simulink model "CompleteEngineModel_turbo"  (R2020a)
settings: Solver=ode23tb  StartTime=0  StopTime=600  MaxStep=0.4  RelTol=1e-6  AbsTol=1e-6  EnableMultiTasking=on
values from neighbouring files (symbols this model uses):
  A_eff_const = inv(A'*A)*A'*B    [Init_Project1.m]
  A_max_wg = 0.035^2/4*pi    (= 0.000962112750162)    [Init_Project1.m]    (also in Project2B.m = 0.000314159265359)
  AFs = EngineMap.airfuel.AFs    [Init_Project1.m]    (also in Project1b.m = 14)
  alpha_REF_manual = 0    [Init_Project1.m]    (also in Project2B.m)
  alphaEND = alphaINI    (= 0)    [Init_Project1.m]
  alphaINI = 0.0    (= 0)    [Init_Project1.m]
  alphaST = 30    [Init_Project1.m]
  Boost_control = 0    [Init_Project1.m]    (also in Project2B.m = 1)
  BSR_max = k(2)    [Project2A.m]
  C_d = x(3)    [Init_Project1.m]
  C_P0 = k(1)    [Project2A.m]
  C_P1 = k(2)    [Project2A.m]
  c_r1 = x(1)    [Init_Project1.m]
  c_r2 = x(2)    [Init_Project1.m]
  c_tc_fric = 1e-6    (= 1e-06)    [Init_Project1.m]    (also in Project2B.m)
  Cd_wg = 0.8    [Init_Project1.m]    (also in Project2B.m = 0.9)
  cp_air = gamma_air*cv_air    [Init_Project1.m]    (also in Project2A.m = 980)
  cp_exh = gamma_exh*cv_exh    [Init_Project1.m]    (also in Project2A.m = 1213.3)
  dP_thrREF = 10e3    (= 10000)    [Project2B.m]
  eta_c_max = k(1)    [Project2A.m]
  eta_t_max = k(1)    [Project2A.m]
  eta_vol_model = Intake_mainfold_const(1) + Intake_mainfold_const(2).*sqrt(p_im) + Intake_mainfold_const(3).*sqrt(N)    [Init_Project1.m]
  etaCmin = min(etaC/2)    [Project2A.m]
  etaTmin = min(turb.etaT)/2    [Project2A.m]
  Exhaust_flow_const = inv(A'*A)*A'*B    [Init_Project1.m]
  FMEP_const = inv(A'*A)*A'*B    [Init_Project1.m]
  Fuel_injection_const = inv(A'*A)*A'*B    [Init_Project1.m]
  gamma_air = EngineMap.airfuel.gamma_air    [Init_Project1.m]    (also in Project2A.m = 1.4)
  gamma_exh = EngineMap.airfuel.gamma_exh    [Init_Project1.m]    (also in Project2A.m = 1.3)
  Intake_mainfold_const = inv(A'*A)*A'*B    [Init_Project1.m]
  J_tc = 2.55e-5    (= 2.55e-05)    [Init_Project1.m]    (also in Project2B.m = 1e-05)
  k_0 = k(1)    [Project2A.m]
  k_1 = k(2)    [Project2A.m]
  KiDriver = 0.02    [Init_Project1.m]    (also in Project2B.m = 0.05)
  KpDriver = 0.04    [Init_Project1.m]    (also in Project2B.m = 0.8)
  KpThr = 1e-6    (= 1e-06)    [Init_Project1.m]    (also in Project2B.m)
  KpWg = 1e-6    (= 1e-06)    [Init_Project1.m]    (also in Project2B.m = 5e-06)
  m_dot_c_Corr_at = k(2)    [Project2A.m]
  m_dot_cCorr_max = k(2)    [Project2A.m]
  n_cyl = EngineMap.engine.n_cyl    [Init_Project1.m]    (also in Project2A.m)
  N_e_manual = 0    [Init_Project1.m]    (also in Project2B.m = 1)
  N_e_step = 1    [Init_Project1.m]    (also in Project2B.m)
  n_r = EngineMap.engine.n_r    [Init_Project1.m]    (also in Project2A.m; Project2B.m = 2)
  NEND = NINI    (= 2000)    [Init_Project1.m]    (also in Project2B.m = 2500)
  NeRampInit = 800    [Init_Project1.m]    (also in Project2B.m)
  NeSlope = 1    [Init_Project1.m]    (also in Project2B.m)
  NeST = 30    [Init_Project1.m]
  NINI = 2000    [Init_Project1.m]    (also in Project2B.m = 2500)
  p01 = comp.p01    [Project2A.m]
  p_amb = max(EngineMap.p_af)    [Init_Project1.m]
  pCref = comp.pCref    [Project2A.m]
  pedEND = 1.0    (= 1)    [Init_Project1.m]    (also in Project2B.m)
  pedINI = 0.2    [Init_Project1.m]    (also in Project2B.m = 0)
  pedPos_manual = 0    [Init_Project1.m]    (also in Project2B.m = 1)
  pedST = 30    [Init_Project1.m]    (also in Project2B.m)
  PiC_at = k(3)    [Project2A.m]
  Psi_max = k(1)    [Project2A.m]
  Q11 = k(4)    [Project2A.m]
  Q12 = k(5)    [Project2A.m]
  Q22 = k(6)    [Project2A.m]
  q_LHV = EngineMap.airfuel.q_LHV    [Init_Project1.m]
  R_air = EngineMap.airfuel.R_air    [Init_Project1.m]
  r_c = EngineMap.engine.r_c    [Init_Project1.m]    (also in Project1b.m = pCylHigh.r_c)
  R_exh = EngineMap.airfuel.R_exh    [Init_Project1.m]
  rComp = dComp/2    (= 0.028)    [Project2A.m]
  rho_air = p_amb/(R_air*T_amb)    [Init_Project1.m]
  rTurb = dTurb/2    (= 0.0261)    [Project2A.m]
  T01 = comp.T01    [Project2A.m]
  T_amb = mean(EngineMap.T_af)    [Init_Project1.m]
  T_bef_thr = EngineMap.T_bef_thr    [Init_Project1.m]
  T_es = EngineMap.T_es    [Init_Project1.m]
  T_ic = mean(T_bef_thr)    [Init_Project1.m]    (also in Project2B.m = T_im)
  T_im = EngineMap.T_im    [Init_Project1.m]    (also in Project1b.m = pCylHigh.T_im)
  tau_d = 0.069    [Init_Project1.m]
  tau_mix = 0.085    [Init_Project1.m]
  tau_th = 0.04    [Init_Project1.m]
  tau_wg = 0.1    [Init_Project1.m]    (also in Project2B.m)
  TCref = comp.TCref    [Project2A.m]
  Temp_const = inv(A'*A)*A'*B    [Init_Project1.m]
  TiThr = 0.1    [Init_Project1.m]    (also in Project2B.m = 0.4)
  TiWg = 4    [Init_Project1.m]    (also in Project2B.m = 7)
  V_D = EngineMap.engine.V_D    [Init_Project1.m]    (also in Project2B.m = n_cyl*V_d)
  V_d = 2*a*pi*B^2/4    [Init_Project1.m]    (also in Project2A.m; Project2B.m = B^2/4*pi*s)
  V_em = EngineMap.engine.V_em    [Init_Project1.m]
  V_es = EngineMap.engine.V_es    [Init_Project1.m]
  V_ic = 10e-3    (= 0.01)    [Init_Project1.m]    (also in Project2B.m)
  V_im = EngineMap.engine.V_im    [Init_Project1.m]
  VehicleArea = 2.0    (= 2)    [Init_Project1.m]
  VehicleMass = 1520    [Init_Project1.m]
  wg_REF_manual = 0    [Init_Project1.m]    (also in Project2B.m)
  wgEND = wgINI    (= 100)    [Init_Project1.m]
  wgINI = 100    [Init_Project1.m]
  wgST = 30    [Init_Project1.m]
  WheelRadius = 0.3    [Init_Project1.m]
undefined symbols (not defined in the file or in its folder): Newton, Raphson, TqEvsNe
libraries: simulink x2
(part 1 of 2)
settings Model: ExtModeTrigMode=oneshot  ExtModeArmWhenConnect=off  ExtModeAutoUpdateStatusClock=off  Creator=peran  LastModifiedBy=David Wiman
settings SolverCC: AutoScaleAbsTol=off
settings DataIOCC: SaveFormat=Array  SignalLoggingSaveFormat=ModelDataLogs  ReturnWorkspaceOutputs=off  SignalLoggingName=sigsOut
settings OptimizationCC: BlockReduction=off  BooleanDataType=off  ExpressionDepthLimit=2147483647  InitFltsAndDblsToZero=on  LifeSpan=inf
settings DebuggingCC: SaveWithParameterizedLinksMsg=none  UnderspecifiedInitializationDetection=Classic  MergeDetectMultiDrivingBlocksExec=none  SignalResolutionControl=TryResolveAllWithWarning  MultiTaskDSMMsg=warning  MultiTaskCondExecSysMsg=none  FcnCallInpInsideContextMsg=warning  StateNameClashWarn=warning  SFUnexpectedBacktrackingDiag=warning  SFNoUnconditionalDefaultTransitionDiag=warning  SFExecutionAtInitializationDiag=none  ArithmeticOperatorsInVariantConditions=warning
settings HardwareCC: ProdBitPerPointer=32  ProdBitPerSizeT=32  ProdBitPerPtrDiffT=32  ProdLargestAtomicFloat=None  ProdIntDivRoundTo=Undefined  ProdEndianess=Unspecified  ProdWordSize=32  ProdHWDeviceType=32-bit Generic  TargetUnknown=on
settings ModelReferenceCC: PropagateSignalLabelsOutOfModel=off
settings SFSimCC: SimUseLocalCustomCode=off  CustomCodeUndefinedFunction=UseInterfaceOnly
settings RTWCC: RTWUseLocalCustomCode=off
settings CodeAppCC: StateflowObjectComments=on
settings GRTTargetCC: TargetFcnLib=ansi_tfl_tmw.mat  TargetLangStandard=C89/C90 (ANSI)  ModelReferenceCompliant=off  CombineOutputUpdateFcns=off  MatFileLogging=off  GRTInterface=on
settings ConfigComp: CovMetricSettings=dw  CovHtmlReporting=on  CovSaveCumulativeToWorkspaceVar=on  CovSaveSingleToWorkspaceVar=on  CovExternalEMLEnable=off

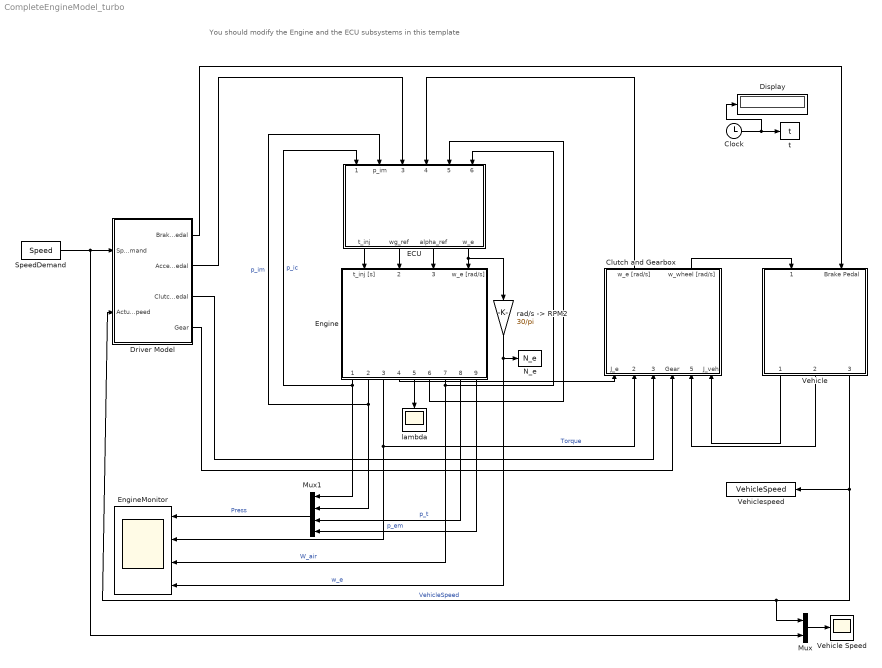
== system CompleteEngineModel_turbo ==
  note: You should modify the Engine and the ECU subsystems in this template
  Clock : Clock
  Clutch and Gearbox : Subsystem
  Display : Display
  Driver Model : Subsystem
  ECU : Subsystem
  Engine : Subsystem
  EngineMonitor : Scope  NumInputPorts=4
  Mux : Mux  Inputs=2
  Mux1 : Mux
  N_e : ToWorkspace  VariableName=N_e  SampleTime=-1
  SpeedDemand : FromWorkspace  VariableName=Speed  ZeroCross=off
  Vehicle : Subsystem
  Vehicle Speed : Scope
  Vehiclespeed : ToWorkspace  VariableName=VehicleSpeed  SampleTime=-1
  lambda : Scope
  "rad/s -> RPM2" : Gain  Gain=30/pi  SaturateOnIntegerOverflow=on  OutDataTypeStr=Inherit: Same as input  ParamDataTypeStr=Inherit: Same as input
  t : ToWorkspace  VariableName=t  SampleTime=-1
  wires:
  Vehicle/1(Vehicle Inertia [kgm^2]) -> Clutch and Gearbox/6(J_veh)
  Vehicle/2(Vehicle Torque [Nm]) -> Clutch and Gearbox/5(Tq_veh [Nm])
  Clutch and Gearbox/2(w_wheel [rad/s]) -> Vehicle/1(Wheel Speed [rad/s])
  Vehicle/3(Vehicle Speed[km/h]) -> Driver Model/2(Actual speed), Mux/1, Vehiclespeed/1  "VehicleSpeed"
  Driver Model/1(Brake Pedal) -> Vehicle/2(Brake Pedal)
  Driver Model/3(Clutch Pedal) -> Clutch and Gearbox/3(Clutch Pedal)
  Driver Model/2(Accelerator Pedal) -> ECU/3(ped_pos)
  Clutch and Gearbox/1(w_e [rad/s]) -> ECU/4(w_e [rad/s])
  SpeedDemand/1 -> Driver Model/1(Speed demand), Mux/2
  Driver Model/4(Gear) -> Clutch and Gearbox/4(Gear)
  Mux/1 -> Vehicle Speed/1
  Clock/1 -> t/1, Display/1
  Engine/7(m_dot_at [kg/s]) -> EngineMonitor/3, ECU/6(m_dot_air [kg/s])  "W_air"
  Engine/6(Lambda Disc) -> ECU/5(lambdaDisc)
  Engine/2(p_im [Pa]) -> Mux1/2, ECU/2(p_im)  "p_im"
  Engine/4(J_e [kgm^2]) -> Clutch and Gearbox/1(J_e)
  Engine/3(M_e [Nm]) -> EngineMonitor/2, Clutch and Gearbox/2(Tq_e [Nm])  "Torque"
  Engine/1(p_bef[Pa]) -> Mux1/1, ECU/1(p_ic [Pa])  "p_ic"
  Mux1/1 -> EngineMonitor/1  "Press"
  Engine/5(Lambda) -> lambda/1
  Engine/8(p_t [Pa]) -> Mux1/3  "p_t"
  Engine/9(p_em  [Pa]) -> Mux1/4  "p_em"
  ECU/4(w_e) -> "rad/s -> RPM2"/1, Engine/4(w_e [rad/s])
  "rad/s -> RPM2"/1 -> EngineMonitor/4, N_e/1  "w_e"
  ECU/2(wg_ref) -> Engine/2(wg_REF [0..1])
  ECU/3(alpha_ref) -> Engine/3(alpha_REF [0..1])
  ECU/1(t_inj) -> Engine/1(t_inj [s])

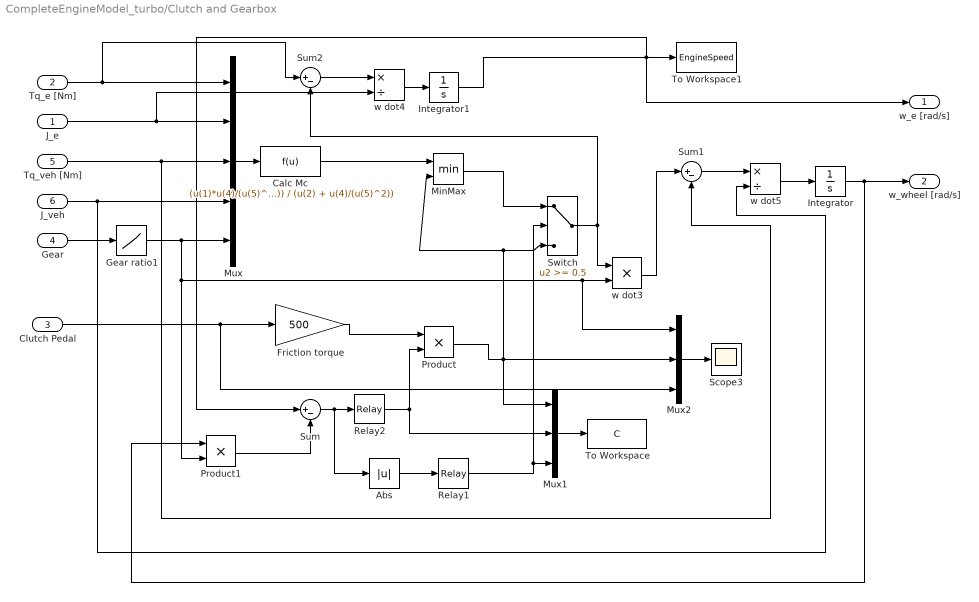
== system CompleteEngineModel_turbo/Clutch and Gearbox ==
  J_e : Inport
  Tq_e [Nm] : Inport  Port=2
  Clutch Pedal : Inport  Port=3
  Gear : Inport  Port=4
  Tq_veh [Nm] : Inport  Port=5
  J_veh : Inport  Port=6
  Abs : Abs  SaturateOnIntegerOverflow=on
  Calc Mc : Fcn  Expr=(u(1)*u(4)/(u(5)^2) + u(2)*u(3)/u(5)) / (u(2) + u(4)/(u(5)^2))
  Friction torque : Gain  Gain=500  SaturateOnIntegerOverflow=on  OutDataTypeStr=Inherit: Same as input  ParamDataTypeStr=Inherit: Same as input
  Gear ratio1 : Lookup  InputValues=[0:5]  Table=[30 16 7.5 4.5 3.2 2.5]  SaturateOnIntegerOverflow=on
  Integrator : Integrator
  Integrator1 : Integrator  InitialCondition=100  LimitOutput=on  LowerSaturationLimit=100
  MinMax : MinMax  Inputs=2  InputSameDT=on  SaturateOnIntegerOverflow=on
  Mux : Mux  Inputs=5
  Mux1 : Mux  Inputs=3
  Mux2 : Mux  Inputs=3
  Product : Product  InputSameDT=on  SaturateOnIntegerOverflow=on  OutDataTypeStr=Inherit: Same as first input
  Product1 : Product  InputSameDT=on  SaturateOnIntegerOverflow=on  OutDataTypeStr=Inherit: Same as first input
  Relay1 : Relay  OnSwitchValue=10  OffSwitchValue=1e-3  OnOutputValue=0  OffOutputValue=1
  Relay2 : Relay  OnSwitchValue=1e-1  OffSwitchValue=-1e-1  OffOutputValue=-1
  Scope3 : Scope
  Sum : Sum  Inputs=|+-  InputSameDT=on  SaturateOnIntegerOverflow=on  OutDataTypeStr=Inherit: Same as first input
  Sum1 : Sum  Inputs=|+-  InputSameDT=on  SaturateOnIntegerOverflow=on  OutDataTypeStr=Inherit: Same as first input
  Sum2 : Sum  Inputs=|+-  InputSameDT=on  SaturateOnIntegerOverflow=on  OutDataTypeStr=Inherit: Same as first input
  Switch : Switch  Threshold=0.5  SaturateOnIntegerOverflow=on  InputSameDT=on
  To Workspace : ToWorkspace  VariableName=C  SaveFormat=Structure With Time  SampleTime=-1
  To Workspace1 : ToWorkspace  VariableName=EngineSpeed  SaveFormat=Structure With Time  SampleTime=-1
  w dot3 : Product  Inputs=**  InputSameDT=on  SaturateOnIntegerOverflow=on  OutDataTypeStr=Inherit: Same as first input
  w dot4 : Product  Inputs=*/  InputSameDT=on  SaturateOnIntegerOverflow=on  OutDataTypeStr=Inherit: Same as first input
  w dot5 : Product  Inputs=*/  InputSameDT=on  SaturateOnIntegerOverflow=on  OutDataTypeStr=Inherit: Same as first input
  w_e [rad/s] : Outport
  w_wheel [rad/s] : Outport  Port=2
  wires:
  Switch/1 -> w dot3/1, Sum2/2
  Relay2/1 -> Mux1/2, Product/2
  Sum/1 -> Relay2/1, Abs/1
  Abs/1 -> Relay1/1
  MinMax/1 -> Switch/1
  Calc Mc/1 -> MinMax/1
  Mux/1 -> Calc Mc/1
  Mux2/1 -> Scope3/1
  Clutch Pedal/1 -> Friction torque/1, Mux2/3
  Tq_e [Nm]/1 -> Mux/1, Sum2/1
  J_e/1 -> Mux/2, w dot4/2
  Sum2/1 -> w dot4/1
  w dot4/1 -> Integrator1/1
  Integrator1/1 -> To Workspace1/1, w_e [rad/s]/1, Sum/1
  Relay1/1 -> Mux1/3, Switch/2
  Mux1/1 -> To Workspace/1
  Product1/1 -> Sum/2
  Product/1 -> MinMax/2, Switch/3, Mux2/2, Mux1/1
  Friction torque/1 -> Product/1
  Gear/1 -> Gear ratio1/1
  Gear ratio1/1 -> Product1/2, w dot3/2, Mux2/1, Mux/5
  w dot5/1 -> Integrator/1
  Sum1/1 -> w dot5/1
  Tq_veh [Nm]/1 -> Mux/3, Sum1/2
  J_veh/1 -> Mux/4, w dot5/2
  Integrator/1 -> w_wheel [rad/s]/1, Product1/1
  w dot3/1 -> Sum1/1

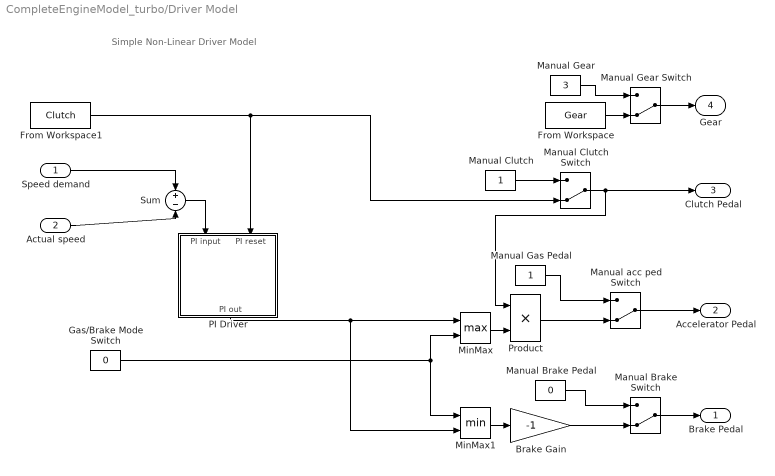
== system CompleteEngineModel_turbo/Driver Model ==
  note: Simple Non-Linear Driver Model
  Speed demand : Inport
  Actual speed : Inport  Port=2
  Brake Gain : Gain  Gain=-1  SaturateOnIntegerOverflow=on  OutDataTypeStr=Inherit: Same as input  ParamDataTypeStr=Inherit: Same as input
  From Workspace : FromWorkspace  VariableName=Gear  ZeroCross=off
  From Workspace1 : FromWorkspace  VariableName=Clutch  ZeroCross=off  OutputAfterFinalValue=Holding final value
  Gas/Brake Mode Switch : Constant  Value=0
  Manual Clutch : Constant
  Manual Gas Pedal : Constant
  Manual Gear : Constant  Value=3
  Manual Brake Pedal : Constant  Value=0
  Manual Brake Switch : ManualSwitch  CurrentSetting=0
  Manual Clutch Switch : ManualSwitch  CurrentSetting=0
  Manual Gear Switch : ManualSwitch  CurrentSetting=0
  Manual acc ped Switch : ManualSwitch  CurrentSetting=0
  MinMax : MinMax  Function=max  Inputs=2  InputSameDT=on  SaturateOnIntegerOverflow=on
  MinMax1 : MinMax  Inputs=2  InputSameDT=on  SaturateOnIntegerOverflow=on
  PI Driver : Subsystem
  Product : Product  InputSameDT=on  SaturateOnIntegerOverflow=on  OutDataTypeStr=Inherit: Same as first input
  Sum : Sum  Inputs=+-  InputSameDT=on  SaturateOnIntegerOverflow=on  OutDataTypeStr=Inherit: Same as first input
  Brake Pedal : Outport
  Accelerator Pedal : Outport  Port=2
  Clutch Pedal : Outport  Port=3
  Gear : Outport  Port=4
  wires:
  Product/1 -> Manual acc ped Switch/2
  MinMax/1 -> Product/2
  Manual acc ped Switch/1 -> Accelerator Pedal/1
  Manual Gas Pedal/1 -> Manual acc ped Switch/1
  Gas/Brake Mode Switch/1 -> MinMax1/1, MinMax/2
  MinMax1/1 -> Brake Gain/1
  PI Driver/1(PI out) -> MinMax1/2, MinMax/1
  From Workspace1/1 -> Manual Clutch Switch/2, PI Driver/2(PI reset)
  Manual Gear/1 -> Manual Gear Switch/1
  From Workspace/1 -> Manual Gear Switch/2
  Manual Gear Switch/1 -> Gear/1
  Manual Clutch/1 -> Manual Clutch Switch/1
  Brake Gain/1 -> Manual Brake Switch/2
  Manual Brake Pedal/1 -> Manual Brake Switch/1
  Manual Brake Switch/1 -> Brake Pedal/1
  Manual Clutch Switch/1 -> Clutch Pedal/1, Product/1
  Speed demand/1 -> Sum/1
  Sum/1 -> PI Driver/1(PI input)
  Actual speed/1 -> Sum/2

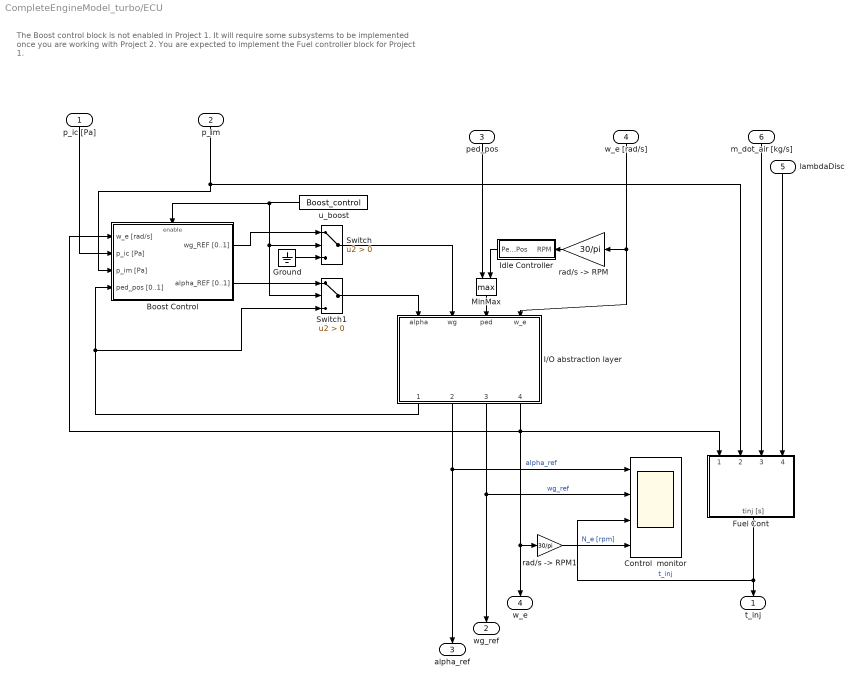
== system CompleteEngineModel_turbo/ECU ==
  note: The Boost control block is not enabled in Project 1. It will require some subsystems to be
      | implemented once you are working with Project 2.
      | You are expected to implement the Fuel controller block for Project 1.
  p_ic [Pa] : Inport
  p_im : Inport  Port=2
  ped_pos : Inport  Port=3
  w_e [rad/s] : Inport  Port=4
  lambdaDisc : Inport  Port=5
  m_dot_air [kg/s] : Inport  Port=6
  Boost Control : Subsystem
  Control  monitor : Scope  NumInputPorts=4
  Fuel Cont : Subsystem
  Ground : Ground
  I/O abstraction layer : Subsystem
  Idle Controller : Subsystem
  MinMax : MinMax  Function=max  Inputs=2  InputSameDT=on  SaturateOnIntegerOverflow=on
  Switch : Switch  Criteria=u2 > Threshold
  Switch1 : Switch  Criteria=u2 > Threshold
  "rad/s -> RPM" : Gain  Gain=30/pi  SaturateOnIntegerOverflow=on  OutDataTypeStr=Inherit: Same as input  ParamDataTypeStr=Inherit: Same as input
  "rad/s -> RPM1" : Gain  Gain=30/pi  SaturateOnIntegerOverflow=on  OutDataTypeStr=Inherit: Same as input  ParamDataTypeStr=Inherit: Same as input
  u_boost : Constant  Value=Boost_control
  t_inj : Outport
  wg_ref : Outport  Port=2
  alpha_ref : Outport  Port=3
  w_e : Outport  Port=4
  wires:
  Idle Controller/1(PedalPos) -> MinMax/2
  MinMax/1 -> I/O abstraction layer/3(ped)
  I/O abstraction layer/4(w_e [rad/s]) -> Boost Control/1("w_e [rad/s] "), Fuel Cont/1(w_e [rad/s]), w_e/1, "rad/s -> RPM1"/1
  w_e [rad/s]/1 -> I/O abstraction layer/4(w_e), "rad/s -> RPM"/1
  m_dot_air [kg/s]/1 -> Fuel Cont/3(m_dot_air [kg/s])
  p_ic [Pa]/1 -> Boost Control/2(p_ic [Pa])
  ped_pos/1 -> MinMax/1
  Fuel Cont/1(tinj [s]) -> Control  monitor/3, t_inj/1  "t_inj"
  I/O abstraction layer/2(alpha_REF [0..1]) -> Control  monitor/1, alpha_ref/1  "alpha_ref"
  I/O abstraction layer/3(wg_REF [0..100]) -> Control  monitor/2, wg_ref/1  "wg_ref"
  lambdaDisc/1 -> Fuel Cont/4(lambdaDisc)
  p_im/1 -> Boost Control/3(p_im [Pa]), Fuel Cont/2(p_im [Pa])
  "rad/s -> RPM"/1 -> Idle Controller/1(RPM)
  I/O abstraction layer/1(pedPos [0..1]) -> Boost Control/4(ped_pos [0..1]), Switch1/3
  u_boost/1 -> Boost Control/Enable, Switch1/2, Switch/2
  Boost Control/2(alpha_REF [0..1]) -> Switch1/1
  Switch1/1 -> I/O abstraction layer/1(alpha)
  Switch/1 -> I/O abstraction layer/2(wg)
  Boost Control/1(wg_REF [0..1]) -> Switch/1
  Ground/1 -> Switch/3
  "rad/s -> RPM1"/1 -> Control  monitor/4  "N_e [rpm]"

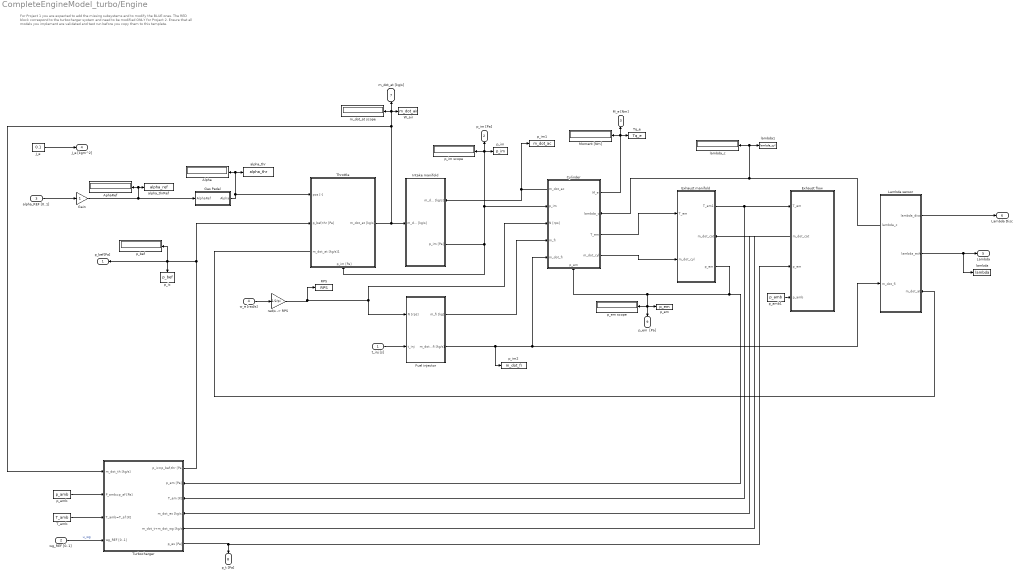
== system CompleteEngineModel_turbo/Engine ==
  note: For Project 1 you are expected to add the missing subsystems and to modify the BLUE ones.
      | The RED block correspond to the turbocharger system and need to be modified ONLY for Project 2.
      | Ensure that all models you implement are validated and test run before you copy them to this template.
  t_inj [s] : Inport
  wg_REF [0..1] : Inport  Port=2
  alpha_REF [0..1] : Inport  Port=3
  w_e [rad/s] : Inport  Port=4
  Alpha : Display
  AphaRef : Display
  Cylinder : Subsystem
      settings: PortSchema="{\"entries\":[{\"content\":{\"sides\":[{\"content\":{\"connectorIds\":[\"Out2\",\"Out3\",\"In1\",\"Out4\"]},\"type\":\"ConnectorPlacement.EquallySpacedRectSide\",\"uuid\":\"c6ff6295-f90b-4986-ac7a-70e0bce22d1f\"},{\"content\":{\"connectorIds\":[\"In3\",\"In4\",\"In5\",\"In6\",\"Out1\"],\"side\":\"RIGHT\"},\"type\":\"ConnectorPlacement.EquallySpacedRectSide\",\"uuid\":\"f8bbf01b-018f-4b58-b1b8-37d8ef2a501b\"},{\"content\":{\"connectorIds\":[\"In2\"],\"side\":\"TOP\"},\"type\":\"ConnectorPlacement.EquallySpacedRectSide\",\"uuid\":\"590f1776-0b6e-490b-9b82-c6a1f0298d63\"},{\"content\":{\"connectorIds\":[],\"side\":\"BOTTOM\"},\"type\":\"ConnectorPlacement.EquallySpacedRectSide\",\"uuid\":\"6fcd95e2-2788-44a0-9284-05f8c21997a1\"}]},\"type\":\"ConnectorPlacement.EquallySpacedConnector\",\"uuid\":\"69b978e9-63f0-4790-9255-9c73cc49e7a8\"}],\"packageUris\":[\"http://schema.mathworks.com/mf0/Connector/19700101\"],\"version\":\"1.0\"}"
  Exhaust flow : Subsystem
      settings: PortSchema="{\"entries\":[{\"content\":{\"sides\":[{\"content\":{\"connectorIds\":[\"In1\",\"Out1\",\"In2\",\"In3\"]},\"type\":\"ConnectorPlacement.EquallySpacedRectSide\",\"uuid\":\"f06335af-0d46-453e-89a7-85820e5b30b4\"},{\"content\":{\"connectorIds\":[],\"side\":\"RIGHT\"},\"type\":\"ConnectorPlacement.EquallySpacedRectSide\",\"uuid\":\"1980f551-ae72-440d-afc1-b2b6b725f391\"},{\"content\":{\"connectorIds\":[],\"side\":\"TOP\"},\"type\":\"ConnectorPlacement.EquallySpacedRectSide\",\"uuid\":\"7f9d811b-4ba7-47b4-9941-e90fdf29edc9\"}]},\"type\":\"ConnectorPlacement.EquallySpacedConnector\",\"uuid\":\"d9ed9e77-87d7-4fb4-9a8b-d019adccfd00\"}],\"packageUris\":[\"http://schema.mathworks.com/mf0/Connector/19700101\"],\"version\":\"1.0\"}"
  Exhaust manifold : Subsystem
      settings: PortSchema="{\"entries\":[{\"content\":{\"sides\":[{\"content\":{\"connectorIds\":[\"In1\",\"In2\"]},\"type\":\"ConnectorPlacement.EquallySpacedRectSide\",\"uuid\":\"ecdbb782-eef7-477e-bb82-5ebf032163a3\"},{\"content\":{\"connectorIds\":[\"Out1\",\"In3\",\"Out2\"],\"side\":\"RIGHT\"},\"type\":\"ConnectorPlacement.EquallySpacedRectSide\",\"uuid\":\"4b5fba5e-4300-4916-aa15-d3f6c61d9689\"},{\"content\":{\"connectorIds\":[],\"side\":\"TOP\"},\"type\":\"ConnectorPlacement.EquallySpacedRectSide\",\"uuid\":\"210fa4c6-63e4-484e-b7fb-4f2899d71e64\"}]},\"type\":\"ConnectorPlacement.EquallySpacedConnector\",\"uuid\":\"ab4f6bcc-96c1-47e6-9038-ce7b6e5d4830\"}],\"packageUris\":[\"http://schema.mathworks.com/mf0/Connector/19700101\"],\"version\":\"1.0\"}"
  Fuel injector : Subsystem
      settings: PortSchema="{\"entries\":[{\"content\":{\"sides\":[{\"content\":{\"connectorIds\":[]},\"type\":\"ConnectorPlacement.EquallySpacedRectSide\",\"uuid\":\"c6ff6295-f90b-4986-ac7a-70e0bce22d1f\"},{\"content\":{\"connectorIds\":[],\"side\":\"RIGHT\"},\"type\":\"ConnectorPlacement.EquallySpacedRectSide\",\"uuid\":\"f8bbf01b-018f-4b58-b1b8-37d8ef2a501b\"},{\"content\":{\"connectorIds\":[\"In1\",\"In2\"],\"side\":\"TOP\"},\"type\":\"ConnectorPlacement.EquallySpacedRectSide\",\"uuid\":\"590f1776-0b6e-490b-9b82-c6a1f0298d63\"},{\"content\":{\"connectorIds\":[\"Out1\",\"Out2\"],\"side\":\"BOTTOM\"},\"type\":\"ConnectorPlacement.EquallySpacedRectSide\",\"uuid\":\"6fcd95e2-2788-44a0-9284-05f8c21997a1\"}]},\"type\":\"ConnectorPlacement.EquallySpacedConnector\",\"uuid\":\"69b978e9-63f0-4790-9255-9c73cc49e7a8\"}],\"packageUris\":[\"http://schema.mathworks.com/mf0/Connector/19700101\"],\"version\":\"1.0\"}"
  Gain : Gain
  Gas Pedal : Subsystem
  Intake manifold : Subsystem
      settings: PortSchema="{\"entries\":[{\"content\":{\"sides\":[{\"content\":{\"connectorIds\":[\"In1\"]},\"type\":\"ConnectorPlacement.EquallySpacedRectSide\",\"uuid\":\"c4e4d620-2bcc-4db0-9055-5904ec1a58a9\"},{\"content\":{\"connectorIds\":[\"In2\",\"Out1\"],\"side\":\"RIGHT\"},\"type\":\"ConnectorPlacement.EquallySpacedRectSide\",\"uuid\":\"7abafa54-675f-4448-8d24-7b3f9f41fe2d\"},{\"content\":{\"connectorIds\":[],\"side\":\"TOP\"},\"type\":\"ConnectorPlacement.EquallySpacedRectSide\",\"uuid\":\"2b3cebc2-f79e-4be9-b6ba-c95bab7e4fe0\"}]},\"type\":\"ConnectorPlacement.EquallySpacedConnector\",\"uuid\":\"07f49e90-8b24-4894-a061-cd1894b00575\"}],\"packageUris\":[\"http://schema.mathworks.com/mf0/Connector/19700101\"],\"version\":\"1.0\"}"
  J_e : Constant  Value=0.1
  Lambda sensor : Subsystem
      settings: PortSchema="{\"entries\":[{\"content\":{\"sides\":[{\"content\":{\"connectorIds\":[\"Out3\",\"In1\"]},\"type\":\"ConnectorPlacement.EquallySpacedRectSide\",\"uuid\":\"d39da2a0-5083-429f-b2a5-f3c55751e588\"},{\"content\":{\"connectorIds\":[\"Out1\",\"Out2\",\"In2\"],\"side\":\"RIGHT\"},\"type\":\"ConnectorPlacement.EquallySpacedRectSide\",\"uuid\":\"7673ed93-c321-42ef-ae67-bddda5587c96\"},{\"content\":{\"connectorIds\":[],\"side\":\"TOP\"},\"type\":\"ConnectorPlacement.EquallySpacedRectSide\",\"uuid\":\"0618fb4e-cce3-4388-971c-f8e6f06df9e4\"}]},\"type\":\"ConnectorPlacement.EquallySpacedConnector\",\"uuid\":\"03a84aa5-1ec4-4792-999b-2db4677b5033\"}],\"packageUris\":[\"http://schema.mathworks.com/mf0/Connector/19700101\"],\"version\":\"1.0\"}"
  Moment [Nm] : Display
  RPS : ToWorkspace  VariableName=RPS  SampleTime=-1
  T_amb : Constant  Value=T_amb
  "Throttle " : Subsystem
      settings: PortSchema="{\"entries\":[{\"content\":{\"sides\":[{\"content\":{\"connectorIds\":[\"Out2\"]},\"type\":\"ConnectorPlacement.EquallySpacedRectSide\",\"uuid\":\"c928f7f6-9f01-47f3-9bc0-46ff39781eb1\"},{\"content\":{\"connectorIds\":[\"In2\",\"In3\",\"Out1\"],\"side\":\"RIGHT\"},\"type\":\"ConnectorPlacement.EquallySpacedRectSide\",\"uuid\":\"8dd06eba-1f93-4a48-ba14-c22296a753f6\"},{\"content\":{\"connectorIds\":[],\"side\":\"TOP\"},\"type\":\"ConnectorPlacement.EquallySpacedRectSide\",\"uuid\":\"bb338683-60ae-4c40-9ad3-c06e2955afea\"},{\"content\":{\"connectorIds\":[\"In1\"],\"side\":\"BOTTOM\"},\"type\":\"ConnectorPlacement.EquallySpacedRectSide\",\"uuid\":\"0777e4e3-014c-463e-89e2-078be8dd0ff9\"}]},\"type\":\"ConnectorPlacement.EquallySpacedConnector\",\"uuid\":\"cbd452b7-e40d-41fa-8c5f-0189a331593c\"}],\"packageUris\":[\"http://schema.mathworks.com/mf0/Connector/19700101\"],\"version\":\"1.0\"}"
  Tq_e : ToWorkspace  VariableName=Tq_e  SampleTime=-1
  Turbocharger : Subsystem
      settings: PortSchema="{\"entries\":[{\"content\":{\"sides\":[{\"content\":{\"connectorIds\":[\"In1\",\"In2\",\"In3\",\"In4\"]},\"type\":\"ConnectorPlacement.EquallySpacedRectSide\",\"uuid\":\"86731332-f34d-46da-85bd-bb4bed14e334\"},{\"content\":{\"connectorIds\":[\"Out1\",\"In5\",\"In6\",\"In7\",\"Out2\",\"Out3\"],\"side\":\"RIGHT\"},\"type\":\"ConnectorPlacement.EquallySpacedRectSide\",\"uuid\":\"d31b5450-3593-487b-907f-2875749d4d92\"},{\"content\":{\"connectorIds\":[],\"side\":\"TOP\"},\"type\":\"ConnectorPlacement.EquallySpacedRectSide\",\"uuid\":\"0bb27454-71b6-4622-a06e-14bed29e19cf\"}]},\"type\":\"ConnectorPlacement.EquallySpacedConnector\",\"uuid\":\"668c2a51-25ad-4723-a90c-4999ba09b381\"}],\"packageUris\":[\"http://schema.mathworks.com/mf0/Connector/19700101\"],\"version\":\"1.0\"}"
  W_air : ToWorkspace  VariableName=m_dot_air  SampleTime=-1
  alpha_thr : ToWorkspace  VariableName=alpha_thr  SampleTime=-1
  alpha_thrRef : ToWorkspace  VariableName=alpha_ref  SampleTime=-1
  lambda : ToWorkspace  VariableName=lambda  SampleTime=-1
  lambda1 : ToWorkspace  VariableName=lambda_cyl  SampleTime=-1
  lambda_c : Display
  m_dot_at scope : Display
  p_amb : Constant  Value=p_amb
  p_amb1 : Constant  Value=p_amb
  p_bef : Display
  p_em : ToWorkspace  VariableName=p_em  SampleTime=-1
  p_em scope : Display
  p_ic : ToWorkspace  VariableName=p_bef  SampleTime=-1
  p_im : ToWorkspace  VariableName=p_im  SampleTime=-1
  p_im scope : Display
  p_im1 : ToWorkspace  VariableName=m_dot_ac  SampleTime=-1
  p_im2 : ToWorkspace  VariableName=m_dot_fi  SampleTime=-1
  "rad/s -> RPS" : Gain  Gain=1/2/pi  SaturateOnIntegerOverflow=on  OutDataTypeStr=Inherit: Same as input  ParamDataTypeStr=Inherit: Same as input
  p_bef[Pa] : Outport
  p_im [Pa] : Outport  Port=2
  M_e [Nm] : Outport  Port=3
  J_e [kgm^2] : Outport  Port=4
  Lambda : Outport  Port=5
  Lambda Disc : Outport  Port=6
  m_dot_at [kg/s] : Outport  Port=7
  p_t [Pa] : Outport  Port=8
  p_em  [Pa] : Outport  Port=9
  wires:
  J_e/1 -> J_e [kgm^2]/1
  Gas Pedal/1(Alpha) -> Alpha/1, alpha_thr/1, "Throttle "/2(pos [-])
  Lambda sensor/2(lambda_exh) -> Lambda/1, lambda/1
  Lambda sensor/1(lambda_disc) -> Lambda Disc/1
  wg_REF [0..1]/1 -> Turbocharger/4(wg_REF [0..1])  "u_wg"
  Turbocharger/3(p_es [Pa]) -> Exhaust flow/2(p_em), p_t [Pa]/1
  Turbocharger/1(p_ic=p_bef,thr [Pa]) -> "Throttle "/3(p_bef,thr [Pa]), p_bef/1, p_ic/1, p_bef[Pa]/1
  Fuel injector/2(m_fi [kg]) -> Cylinder/4(m_fi)
  Fuel injector/1(m_dot_fi [kg/s]) -> p_im2/1, Lambda sensor/1(m_dot_fi), Cylinder/3(m_dot_fi)
  Exhaust flow/1(m_dot_cat) -> Turbocharger/7(m_dot_es [kg/s])
  p_amb1/1 -> Exhaust flow/3(p_amb)
  Cylinder/1(m_dot_ac) -> p_im1/1, Intake manifold/2(m_dot_ac [kg/s])
  Gain/1 -> AphaRef/1, alpha_thrRef/1, Gas Pedal/1(AlphaRef)
  "rad/s -> RPS"/1 -> RPS/1, Fuel injector/2(N [rps]), Cylinder/5(N [rps])
  t_inj [s]/1 -> Fuel injector/1(t_inj)
  Intake manifold/1(p_im [Pa]) -> p_im/1, p_im scope/1, p_im [Pa]/1, Cylinder/6(p_im), "Throttle "/1(p_im [Pa])
  "Throttle "/2(m_dot_at [kg/s]) -> W_air/1, m_dot_at scope/1, m_dot_at [kg/s]/1, Turbocharger/1(m_dot_th [kg/s]), Intake manifold/1(m_dot_at [kg/s])
  Cylinder/4(M_e) -> Moment [Nm]/1, M_e [Nm]/1, Tq_e/1
  Cylinder/2(m_dot_cyl) -> Exhaust manifold/2(m_dot_cyl)
  Cylinder/3(T_em) -> Exhaust manifold/1(T_em)
  Exhaust manifold/1(T_em1) -> Turbocharger/6(T_em [K]), Exhaust flow/1(T_em)
  Exhaust manifold/2(p_em) -> Turbocharger/5(p_em [Pa]), p_em/1, p_em scope/1, p_em  [Pa]/1, Cylinder/2(p_em)
  Lambda sensor/3(lambda_c) -> lambda1/1, lambda_c/1, Cylinder/1(lambda_c)
  "Throttle "/1(m_dot_at [kg/s]1) -> Lambda sensor/2(m_dot_at)
  alpha_REF [0..1]/1 -> Gain/1
  w_e [rad/s]/1 -> "rad/s -> RPS"/1
  T_amb/1 -> Turbocharger/3(T_amb=T_af [K])
  p_amb/1 -> Turbocharger/2("P_amb=p_af [Pa] ")
  Turbocharger/2(m_dot_t+m_dot_wg [kg/s]) -> Exhaust manifold/3(m_dot_cat)

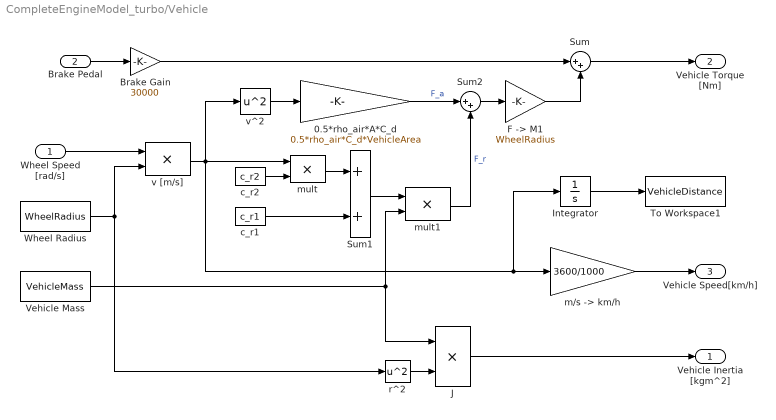
== system CompleteEngineModel_turbo/Vehicle ==
  Wheel Speed [rad/s] : Inport
  Brake Pedal : Inport  Port=2
  0.5*rho_air*A*C_d : Gain  Gain=0.5*rho_air*C_d*VehicleArea  SaturateOnIntegerOverflow=on  OutDataTypeStr=Inherit: Same as input  ParamDataTypeStr=Inherit: Same as input
  Brake Gain : Gain  Gain=30000  SaturateOnIntegerOverflow=on  OutDataTypeStr=Inherit: Same as input  ParamDataTypeStr=Inherit: Same as input
  "F -> M1" : Gain  Gain=WheelRadius  SaturateOnIntegerOverflow=on  OutDataTypeStr=Inherit: Same as input  ParamDataTypeStr=Inherit: Same as input
  Integrator : Integrator
  J : Product  SaturateOnIntegerOverflow=on  OutDataTypeStr=Inherit: Same as first input
  Sum : Sum  Inputs=|++  SaturateOnIntegerOverflow=on
  Sum1 : Sum  SaturateOnIntegerOverflow=on
  Sum2 : Sum  Inputs=|++  SaturateOnIntegerOverflow=on
  To Workspace1 : ToWorkspace  VariableName=VehicleDistance  SampleTime=-1
  Vehicle Mass : Constant  Value=VehicleMass
  Wheel Radius : Constant  Value=WheelRadius
  c_r1 : Constant  Value=c_r1
  c_r2 : Constant  Value=c_r2
  "m/s -> km/h" : Gain  Gain=3600/1000  SaturateOnIntegerOverflow=on  OutDataTypeStr=Inherit: Same as input  ParamDataTypeStr=Inherit: Same as input
  mult : Product  SaturateOnIntegerOverflow=on  OutDataTypeStr=Inherit: Same as first input
  mult1 : Product  SaturateOnIntegerOverflow=on  OutDataTypeStr=Inherit: Same as first input
  r^2 : Math  Operator=square  SignedPower=on  SaturateOnIntegerOverflow=on
  v [m/s] : Product  SaturateOnIntegerOverflow=on  OutDataTypeStr=Inherit: Same as first input
  v^2 : Math  Operator=square  SignedPower=on  SaturateOnIntegerOverflow=on
  Vehicle Inertia [kgm^2] : Outport
  Vehicle Torque [Nm] : Outport  Port=2
  Vehicle Speed[km/h] : Outport  Port=3
  wires:
  Brake Pedal/1 -> Brake Gain/1
  Wheel Radius/1 -> v [m/s]/2, r^2/1
  v [m/s]/1 -> Integrator/1, "m/s -> km/h"/1, mult/1, v^2/1
  "m/s -> km/h"/1 -> Vehicle Speed[km/h]/1
  Brake Gain/1 -> Sum/1
  Sum/1 -> Vehicle Torque [Nm]/1
  r^2/1 -> J/2
  Vehicle Mass/1 -> mult1/2, J/1
  J/1 -> Vehicle Inertia [kgm^2]/1
  Integrator/1 -> To Workspace1/1
  Wheel Speed [rad/s]/1 -> v [m/s]/1
  c_r2/1 -> mult/2
  mult/1 -> Sum1/1
  c_r1/1 -> Sum1/2
  Sum1/1 -> mult1/1
  mult1/1 -> Sum2/2  "F_r"
  v^2/1 -> 0.5*rho_air*A*C_d/1
  0.5*rho_air*A*C_d/1 -> Sum2/1  "F_a"
  Sum2/1 -> "F -> M1"/1
  "F -> M1"/1 -> Sum/2

== system CompleteEngineModel_turbo/Driver Model/PI Driver ==
  PI input : Inport
  PI reset : Inport  Port=2
  Integrator : Integrator  ExternalReset=either  LimitOutput=on  UpperSaturationLimit=30  LowerSaturationLimit=0
  Ki : Gain  Gain=KiDriver  SaturateOnIntegerOverflow=on  OutDataTypeStr=Inherit: Same as input  ParamDataTypeStr=Inherit: Same as input
  Kp : Gain  Gain=KpDriver  SaturateOnIntegerOverflow=on  OutDataTypeStr=Inherit: Same as input  ParamDataTypeStr=Inherit: Same as input
  Saturation : Saturate  UpperLimit=1  LowerLimit=-1
  Sum : Sum  Inputs=|++  InputSameDT=on  SaturateOnIntegerOverflow=on  OutDataTypeStr=Inherit: Same as first input
  PI out : Outport
  wires:
  PI input/1 -> Kp/1, Integrator/1
  Integrator/1 -> Ki/1
  Ki/1 -> Sum/2
  Sum/1 -> Saturation/1
  Saturation/1 -> PI out/1
  PI reset/1 -> Integrator/2
  Kp/1 -> Sum/1

== system CompleteEngineModel_turbo/ECU/Boost Control ==
  note: For Project 2 , the diver gas pedal interpretation and the throttle feed forward blocks need to be implemented.
  "w_e [rad/s] " : Inport
  p_ic [Pa] : Inport  Port=2
  p_im [Pa] : Inport  Port=3
  ped_pos [0..1] : Inport  Port=4
  Enable : EnablePort
  Constant : Constant  Value=0
  Constant1 : Constant
  Driver gas pedal interpretation : Subsystem
  Subtract1 : Sum
  Throttle saturation [0..1] : Saturate  UpperLimit=1  LowerLimit=0
  "Throttle Feed Forward " : Subsystem
  Throttle Feedback including anti-windup : Subsystem
  Waste-gate saturation [0..1] : Saturate  UpperLimit=1  LowerLimit=0
  Waste-gate Feedback including anti-windup1 : Subsystem
  "rad/s -> rpm" : Gain  Gain=30/pi  SaturateOnIntegerOverflow=on  OutDataTypeStr=Inherit: Same as input  ParamDataTypeStr=Inherit: Same as input
  thr_feedback_switch : ManualSwitch
  wg_feedback_switch : ManualSwitch
  wg_REF [0..1] : Outport
  alpha_REF [0..1] : Outport  Port=2
  wires:
  "Throttle Feed Forward "/1(alpha_thrFF [0..1]) -> Subtract1/1
  Throttle Feedback including anti-windup/1(alpha_thrFB [0..1]) -> thr_feedback_switch/1
  Subtract1/1 -> Throttle saturation [0..1]/1, Throttle Feedback including anti-windup/4(alpha_thrREF [0..1])
  "rad/s -> rpm"/1 -> "Throttle Feed Forward "/2(N_e [rpm]), Driver gas pedal interpretation/2(N_e [rpm])
  Throttle saturation [0..1]/1 -> alpha_REF [0..1]/1, Throttle Feedback including anti-windup/3(alpha_thrREFsat [0..1])
  Waste-gate saturation [0..1]/1 -> wg_REF [0..1]/1, Waste-gate Feedback including anti-windup1/3(wgREFsat [0..1])
  "w_e [rad/s] "/1 -> "rad/s -> rpm"/1
  p_ic [Pa]/1 -> Waste-gate Feedback including anti-windup1/2(p_icACT [Pa]), "Throttle Feed Forward "/3(p_icACT [Pa])
  p_im [Pa]/1 -> Throttle Feedback including anti-windup/2(p_imACT [Pa])
  Driver gas pedal interpretation/1(p_im_ref) -> "Throttle Feed Forward "/1(p_imREF [Pa]), Throttle Feedback including anti-windup/1(p_imREF [Pa])
  Driver gas pedal interpretation/2(p_ic_ref) -> Waste-gate Feedback including anti-windup1/1(p_icREF [Pa])
  Constant/1 -> thr_feedback_switch/2
  thr_feedback_switch/1 -> Subtract1/2
  ped_pos [0..1]/1 -> Driver gas pedal interpretation/1(ped_pos [0..1])
  Waste-gate Feedback including anti-windup1/1(wgFB [0..1]) -> wg_feedback_switch/1, Waste-gate Feedback including anti-windup1/4(wgREF [0..1])
  Constant1/1 -> wg_feedback_switch/2
  wg_feedback_switch/1 -> Waste-gate saturation [0..1]/1

== system CompleteEngineModel_turbo/ECU/Fuel Cont ==
  note: You have to implement here your fuel controller
  w_e [rad/s] : Inport
  p_im [Pa] : Inport  Port=2
  m_dot_air [kg/s] : Inport  Port=3
  lambdaDisc : Inport  Port=4
  Constant1 : Constant
  Divide1 : Product  Inputs=*/
  Gain : Gain  Gain=1/AFs
  Gain2 : Gain  Gain=n_r/(n_cyl*Fuel_injection_const(1))
  PID Controller : simulink/Continuous/PID Controller  Controller=PI  Form=Parallel  TimeDomain=Continuous-time  UseExternalTs=off  SampleTime=-1  IntegratorMethod=Forward Euler  FilterMethod=Forward Euler  ControllerParametersSource=internal  P=0.069*0.1/2  I=0.1  D=0.1  UseFilter=on  N=100  TunerSelectOption=Transfer Function Based (PID Tuner App)  InitialConditionSource=internal  InitialConditionForIntegrator=0  InitialConditionForFilter=0  DifferentiatorICPrevScaledInput=0  ExternalReset=none  TrackingMode=off  Kt=1  LimitOutput=off  UpperSaturationLimit=0.5  LowerSaturationLimit=-0.5  LinearizeAsGain=on  AntiWindupMode=none  Kb=1  POutMin=[]  POutMax=[]  IOutMin=[]  IOutMax=[]  DOutMin=[]  DOutMax=[]  NOutMin=[]  NOutMax=[]  SumOutMin=[]  SumOutMax=[]  SaturationOutMin=[]  SaturationOutMax=[]  PParamMin=[]  PParamMax=[]  IParamMin=[]  IParamMax=[]  DParamMin=[]  DParamMax=[]  NParamMin=[]  NParamMax=[]  KbParamMin=[]  KbParamMax=[]  KtParamMin=[]  KtParamMax=[]  KbOutMin=[]  KbOutMax=[]  KtOutMin=[]  KtOutMax=[]  IntegratorOutMin=[]  IntegratorOutMax=[]  FilterOutMin=[]  FilterOutMax=[]  SumI1OutMin=[]  SumI1OutMax=[]  SumI2OutMin=[]  SumI2OutMax=[]  SumI3OutMin=[]  SumI3OutMax=[]  SumI4OutMin=[]  SumI4OutMax=[]  SumDOutMin=[]  SumDOutMax=[]  DifferentiatorOutMin=[]  DifferentiatorOutMax=[]  FilterDiffOutCoefMin=[]  FilterDiffOutCoefMax=[]  ReciprocalOutMin=[]  ReciprocalOutMax=[]  SumDenOutMin=[]  SumDenOutMax=[]  SumNumOutMin=[]  SumNumOutMax=[]  DivideOutMin=[]  DivideOutMax=[]  UdiffTsProdOutMin=[]  UdiffTsProdOutMax=[]  NTsProdOutMin=[]  NTsProdOutMax=[]  UintegralTsProdOutMin=[]  UintegralTsProdOutMax=[]  UngainTsProdOutMin=[]  UngainTsProdOutMax=[]  IntegratorContinuousStateAttributes=''  IntegratorStateMustResolveToSignalObject=off  IntegratorRTWStateStorageClass=Auto  FilterContinuousStateAttributes=''  FilterStateMustResolveToSignalObject=off  FilterRTWStateStorageClass=Auto  ParallelPVariant=InternalParameters  IdealPVariant=Disabled  IVariant=InternalParameters  DVariant=Disabled  IntegratorVariant=Continuous  SatVariant=Disabled  AWVariant=Passthrough  PCopyVariant=Disabled  TRVariant=Disabled  FdbkBlocksVariant=Forward  IdealPFdbkVariant=Disabled  SatFdbkVariant=Disabled  DerivativeFilterVariant=Disabled  NVariant=Disabled  NCopyVariant=Disabled_SignalSpec  FilterICVariant=Disabled  IntegratorICVariant=InternalICs  ExternalResetVariant=Disabled  TRSumVariant=Passthrough  SumFdbkVariant=Disabled  SumVariant=Sum_PI  TsampFilterVariant=InternalTs  TsampNgainVariant=Passthrough  TsampIntegralVariant=Passthrough
  Product : Product
  Sum : Sum  Inputs=|++
  Sum1 : Sum  Inputs=|++
  Terminator1 : Terminator
  m_dot_ac_system : Subsystem
  "rad/s -> RPS" : Gain  Gain=1/2/pi  SaturateOnIntegerOverflow=on  OutDataTypeStr=Inherit: Same as input  ParamDataTypeStr=Inherit: Same as input
  t_0 : Constant  Value=Fuel_injection_const(2)
  tinj [s] : Outport
  wires:
  p_im [Pa]/1 -> m_dot_ac_system/1(p_im)
  lambdaDisc/1 -> PID Controller/1
  m_dot_ac_system/1(m_dot_ac) -> Gain/1
  Gain/1 -> Product/1
  m_dot_air [kg/s]/1 -> Terminator1/1
  Gain2/1 -> Divide1/1
  Divide1/1 -> Sum1/1
  t_0/1 -> Sum1/2
  Sum1/1 -> tinj [s]/1
  "rad/s -> RPS"/1 -> Divide1/2, m_dot_ac_system/2(N)
  PID Controller/1 -> Sum/1
  Constant1/1 -> Sum/2
  Product/1 -> Gain2/1
  w_e [rad/s]/1 -> "rad/s -> RPS"/1
  Sum/1 -> Product/2  "F_fc"

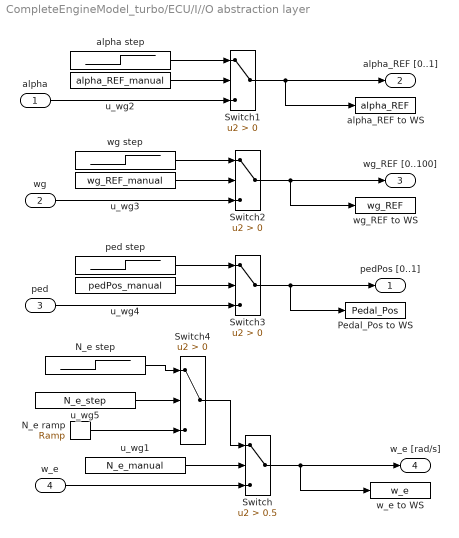
== system CompleteEngineModel_turbo/ECU/I//O abstraction layer ==
  alpha : Inport
  wg : Inport  Port=2
  ped : Inport  Port=3
  w_e : Inport  Port=4
  N_e ramp : simulink/Sources/Ramp  slope=NeSlope*pi/30  start=NeStartTime  InitialOutput=NeRampInit*pi/30
  N_e step : Step  Time=NeST  Before=NINI*pi/30  After=NEND*pi/30  SampleTime=0
  Pedal_Pos to WS : ToWorkspace  VariableName=Pedal_Pos  SampleTime=-1
  Switch : Switch  Criteria=u2 > Threshold  Threshold=0.5
  Switch{1..4} (4 alike) : Switch  Criteria=u2 > Threshold
  alpha step : Step  Time=alphaST  Before=alphaINI  After=alphaEND  SampleTime=0
  alpha_REF to WS : ToWorkspace  VariableName=alpha_REF  SampleTime=-1
  ped step : Step  Time=pedST  Before=pedINI  After=pedEND  SampleTime=0
  u_wg1 : Constant  Value=N_e_manual
  u_wg2 : Constant  Value=alpha_REF_manual
  u_wg3 : Constant  Value=wg_REF_manual
  u_wg4 : Constant  Value=pedPos_manual
  u_wg5 : Constant  Value=N_e_step
  w_e to WS : ToWorkspace  VariableName=w_e  SampleTime=-1
  wg step : Step  Time=wgST  Before=wgINI  After=wgEND  SampleTime=0
  wg_REF to WS : ToWorkspace  VariableName=wg_REF  SampleTime=-1
  pedPos [0..1] : Outport
  alpha_REF [0..1] : Outport  Port=2
  wg_REF [0..100] : Outport  Port=3
  w_e [rad/s] : Outport  Port=4
  wires:
  Switch/1 -> w_e [rad/s]/1, w_e to WS/1
  u_wg1/1 -> Switch/2
  w_e/1 -> Switch/3
  Switch1/1 -> alpha_REF [0..1]/1, alpha_REF to WS/1
  alpha step/1 -> Switch1/1
  u_wg2/1 -> Switch1/2
  alpha/1 -> Switch1/3
  Switch2/1 -> wg_REF [0..100]/1, wg_REF to WS/1
  wg step/1 -> Switch2/1
  u_wg3/1 -> Switch2/2
  wg/1 -> Switch2/3
  Switch3/1 -> pedPos [0..1]/1, Pedal_Pos to WS/1
  ped step/1 -> Switch3/1
  u_wg4/1 -> Switch3/2
  ped/1 -> Switch3/3
  N_e step/1 -> Switch4/1
  Switch4/1 -> Switch/1
  N_e ramp/1 -> Switch4/3
  u_wg5/1 -> Switch4/2

== system CompleteEngineModel_turbo/ECU/Idle Controller ==
  RPM : Inport
  Constant : Constant  Value=800
  Gain : Gain  Gain=1/40000  SaturateOnIntegerOverflow=on  OutDataTypeStr=Inherit: Same as input  ParamDataTypeStr=Inherit: Same as input
  Saturation : Saturate  UpperLimit=1  LowerLimit=0
  Sum : Sum  Inputs=-+  InputSameDT=on  SaturateOnIntegerOverflow=on  OutDataTypeStr=Inherit: Same as first input
  PedalPos : Outport
  wires:
  RPM/1 -> Sum/1
  Constant/1 -> Sum/2
  Saturation/1 -> PedalPos/1
  Gain/1 -> Saturation/1
  Sum/1 -> Gain/1

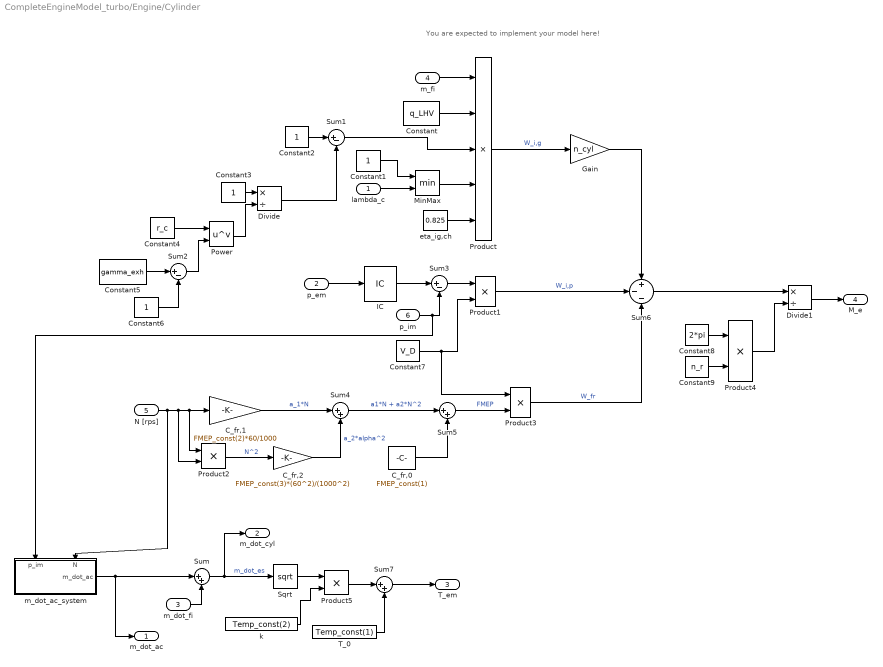
== system CompleteEngineModel_turbo/Engine/Cylinder ==
  note: You are expected to implement your model here!
  lambda_c : Inport
  p_em : Inport  Port=2
  m_dot_fi : Inport  Port=3
  m_fi : Inport  Port=4
  N [rps] : Inport  Port=5
  p_im : Inport  Port=6
  C_fr,0 : Constant  Value=FMEP_const(1)
  C_fr,1 : Gain  Gain=FMEP_const(2)*60/1000
  C_fr,2 : Gain  Gain=FMEP_const(3)*(60^2)/(1000^2)
  Constant : Constant  Value=q_LHV
  Constant{1..3,6} (4 alike) : Constant
  Constant4 : Constant  Value=r_c
  Constant5 : Constant  Value=gamma_exh
  Constant7 : Constant  Value=V_D
  Constant8 : Constant  Value=2*pi
  Constant9 : Constant  Value=n_r
  Divide : Product  Inputs=*/
  Divide1 : Product  Inputs=*/
  Gain : Gain  Gain=n_cyl
  IC : InitialCondition  Value=1.1e5
  MinMax : MinMax  Inputs=2
  Power : Math  Operator=pow  SaturateOnIntegerOverflow=on
  Product : Product  Inputs=5
  Product{1..5} (5 alike) : Product
  Sqrt : Sqrt  SaturateOnIntegerOverflow=on
  Sum{,4..5,7} (4 alike) : Sum  Inputs=|++
  Sum1 : Sum  Inputs=|+-
  Sum2 : Sum  Inputs=|+-
  Sum3 : Sum  Inputs=|+-
  Sum6 : Sum  Inputs=+--
  T_0 : Constant  Value=Temp_const(1)
  eta_ig,ch : Constant  Value=0.825
  k : Constant  Value=Temp_const(2)
  m_dot_ac_system : Subsystem
      settings: PortSchema="{\"entries\":[{\"content\":{\"sides\":[{\"content\":{\"connectorIds\":[]},\"type\":\"ConnectorPlacement.EquallySpacedRectSide\",\"uuid\":\"ecdbb782-eef7-477e-bb82-5ebf032163a3\"},{\"content\":{\"connectorIds\":[\"Out1\"],\"side\":\"RIGHT\"},\"type\":\"ConnectorPlacement.EquallySpacedRectSide\",\"uuid\":\"4b5fba5e-4300-4916-aa15-d3f6c61d9689\"},{\"content\":{\"connectorIds\":[\"In1\",\"In2\"],\"side\":\"TOP\"},\"type\":\"ConnectorPlacement.EquallySpacedRectSide\",\"uuid\":\"210fa4c6-63e4-484e-b7fb-4f2899d71e64\"}]},\"type\":\"ConnectorPlacement.EquallySpacedConnector\",\"uuid\":\"ab4f6bcc-96c1-47e6-9038-ce7b6e5d4830\"}],\"packageUris\":[\"http://schema.mathworks.com/mf0/Connector/19700101\"],\"version\":\"1.0\"}"
  m_dot_ac : Outport
  m_dot_cyl : Outport  Port=2
  T_em : Outport  Port=3
  M_e : Outport  Port=4
  wires:
  m_dot_ac_system/1(m_dot_ac) -> m_dot_ac/1, Sum/1
  m_dot_fi/1 -> Sum/2
  Sum/1 -> m_dot_cyl/1, Sqrt/1  "m_dot_es"
  m_fi/1 -> Product/1
  Constant/1 -> Product/2
  MinMax/1 -> Product/4
  lambda_c/1 -> MinMax/2
  Constant1/1 -> MinMax/1
  eta_ig,ch/1 -> Product/5
  Constant2/1 -> Sum1/1
  Constant3/1 -> Divide/1
  Constant4/1 -> Power/1
  Constant5/1 -> Sum2/1
  Constant6/1 -> Sum2/2
  Sum2/1 -> Power/2
  Power/1 -> Divide/2
  Divide/1 -> Sum1/2
  Sum1/1 -> Product/3
  Product/1 -> Gain/1  "W_i,g"
  p_em/1 -> IC/1
  p_im/1 -> m_dot_ac_system/1(p_im), Sum3/2
  Sum3/1 -> Product1/1
  Constant7/1 -> Product3/1, Product1/2
  Product1/1 -> Sum6/2  "W_i,p"
  Sum4/1 -> Sum5/1  "a1*N + a2*N^2"
  C_fr,1/1 -> Sum4/1  "a_1*N"
  Sum5/1 -> Product3/2  "FMEP"
  Product2/1 -> C_fr,2/1  "N^2"
  N [rps]/1 -> m_dot_ac_system/2(N), Product2/2, Product2/1, C_fr,1/1
  C_fr,2/1 -> Sum4/2  "a_2*alpha^2"
  C_fr,0/1 -> Sum5/2
  Product3/1 -> Sum6/3  "W_fr"
  Sum6/1 -> Divide1/1
  Constant8/1 -> Product4/1
  Constant9/1 -> Product4/2
  Product4/1 -> Divide1/2
  Sqrt/1 -> Product5/1
  k/1 -> Product5/2
  Product5/1 -> Sum7/1
  T_0/1 -> Sum7/2
  Sum7/1 -> T_em/1
  IC/1 -> Sum3/1
  Divide1/1 -> M_e/1
  Gain/1 -> Sum6/1

== system CompleteEngineModel_turbo/Engine/Exhaust flow ==
  note: You are expected to implement your model here!
  T_em : Inport
  p_em : Inport  Port=2
  p_amb : Inport  Port=3
  Divide1 : Product  Inputs=*/
  Gain : Gain  Gain=R_exh
  Gain1 : Gain  Gain=Exhaust_flow_const
  IC : InitialCondition  Value=1.1e5
  Product2 : Product
  Saturation : Saturate  UpperLimit=1000000  LowerLimit=0
  Sqrt : Sqrt  SaturateOnIntegerOverflow=on
  Sum1 : Sum  Inputs=|+-
  m_dot_cat : Outport
  wires:
  p_em/1 -> IC/1
  p_amb/1 -> Sum1/2
  Sum1/1 -> Saturation/1
  Divide1/1 -> Product2/1
  Saturation/1 -> Product2/2
  Product2/1 -> Sqrt/1
  T_em/1 -> Gain/1
  Gain/1 -> Divide1/2
  Sqrt/1 -> Gain1/1
  Gain1/1 -> m_dot_cat/1
  IC/1 -> Divide1/1, Sum1/1

== system CompleteEngineModel_turbo/Engine/Exhaust manifold ==
  note: You are expected to implement your model here!
  T_em : Inport
  m_dot_cyl : Inport  Port=2
  m_dot_cat : Inport  Port=3
  Gain : Gain  Gain=R_exh/V_em
  IC : InitialCondition  Value=1.1e5
  Integrator : Integrator  InitialCondition=1.1e5
  Product3 : Product
  Sum1 : Sum  Inputs=|+-
  T_em1 : Outport
  p_em : Outport  Port=2
  wires:
  m_dot_cyl/1 -> Sum1/1
  Sum1/1 -> Product3/1
  T_em/1 -> T_em1/1, Product3/2
  Product3/1 -> Gain/1
  m_dot_cat/1 -> Sum1/2
  Gain/1 -> Integrator/1
  Integrator/1 -> IC/1
  IC/1 -> p_em/1

== system CompleteEngineModel_turbo/Engine/Fuel injector ==
  note: You are expected to implement your model here!
  t_inj : Inport
  N [rps] : Inport  Port=2
  Constant : Constant  Value=n_cyl
  Constant1 : Constant  Value=n_r
  Divide : Product  Inputs=*/
  Product : Product
  Product1 : Product  Inputs=3
  Sum : Sum  Inputs=|+-
  c_fi : Constant  Value=Fuel_injection_const(1)
  t_0 : Constant  Value=Fuel_injection_const(2)
  m_dot_fi [kg/s] : Outport
  m_fi [kg] : Outport  Port=2
  wires:
  N [rps]/1 -> Product1/1
  c_fi/1 -> Product/1
  t_0/1 -> Sum/2
  Sum/1 -> Product/2
  Constant1/1 -> Divide/2
  Divide/1 -> m_dot_fi [kg/s]/1
  Constant/1 -> Product1/2
  Product1/1 -> Divide/1
  t_inj/1 -> Sum/1
  Product/1 -> m_fi [kg]/1, Product1/3

== system CompleteEngineModel_turbo/Engine/Gas Pedal ==
  note: You are expected to implement your model here!
  AlphaRef : Inport
  Gain : Gain  Gain=1/tau_th
  Integrator : Integrator
  Sum : Sum  Inputs=|+-
  Alpha : Outport
  wires:
  Sum/1 -> Gain/1
  Gain/1 -> Integrator/1  "alpha_dot"
  AlphaRef/1 -> Sum/1
  Integrator/1 -> Alpha/1, Sum/2

== system CompleteEngineModel_turbo/Engine/Intake manifold ==
  note: You are expected to implement your model here!
  m_dot_at [kg/s] : Inport
  m_dot_ac [kg/s] : Inport  Port=2
  Divide : Product  Inputs=*/
  Integrator : Integrator  InitialCondition=15818
  Product : Product
  Product1 : Product
  R : Constant  Value=R_air
  Sum : Sum  Inputs=|+-  SaturateOnIntegerOverflow=on
  T_im : Constant  Value=mean(T_im)
  V_im : Constant  Value=V_im
  p_im [Pa] : Outport
  wires:
  m_dot_ac [kg/s]/1 -> Sum/2
  m_dot_at [kg/s]/1 -> Sum/1
  Product/1 -> Product1/2
  Divide/1 -> Integrator/1
  T_im/1 -> Product/1
  Product1/1 -> Divide/1
  R/1 -> Product/2
  Sum/1 -> Product1/1
  V_im/1 -> Divide/2
  Integrator/1 -> p_im [Pa]/1

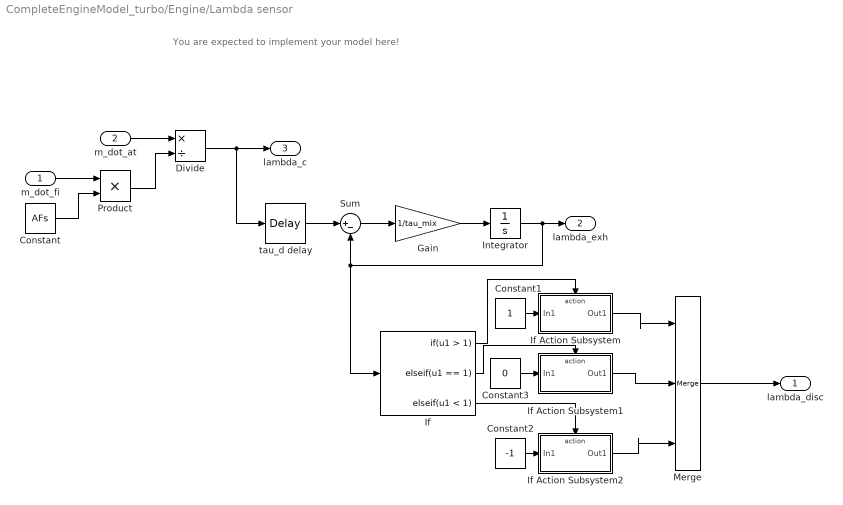
== system CompleteEngineModel_turbo/Engine/Lambda sensor ==
  note: You are expected to implement your model here!
  m_dot_fi : Inport
  m_dot_at : Inport  Port=2
  Constant : Constant  Value=AFs
  Constant1 : Constant
  Constant2 : Constant  Value=-1
  Constant3 : Constant  Value=0
  Divide : Product  Inputs=*/
  Gain : Gain  Gain=1/tau_mix
  If : If  IfExpression=u1 > 1  ElseIfExpressions=u1 == 1, u1 < 1  ShowElse=off
  If Action Subsystem : Subsystem  TreatAsAtomicUnit=on
  If Action Subsystem1 : Subsystem  TreatAsAtomicUnit=on
  If Action Subsystem2 : Subsystem  TreatAsAtomicUnit=on
  Integrator : Integrator  InitialCondition=1
  Merge : Merge  Inputs=3
  Product : Product
  Sum : Sum  Inputs=|+-
  tau_d delay : TransportDelay  DelayTime=tau_d
  lambda_disc : Outport
  lambda_exh : Outport  Port=2
  lambda_c : Outport  Port=3
  wires:
  m_dot_fi/1 -> Product/1
  Constant/1 -> Product/2
  m_dot_at/1 -> Divide/1
  Product/1 -> Divide/2
  Divide/1 -> tau_d delay/1, lambda_c/1
  tau_d delay/1 -> Sum/1
  Sum/1 -> Gain/1
  Gain/1 -> Integrator/1
  Integrator/1 -> If/1, Sum/2, lambda_exh/1
  Merge/1 -> lambda_disc/1
  If/1 -> If Action Subsystem/Action
  Constant1/1 -> If Action Subsystem/1(In1)
  If/3 -> If Action Subsystem2/Action
  Constant2/1 -> If Action Subsystem2/1(In1)
  If/2 -> If Action Subsystem1/Action
  Constant3/1 -> If Action Subsystem1/1(In1)
  If Action Subsystem/1(Out1) -> Merge/1
  If Action Subsystem1/1(Out1) -> Merge/2
  If Action Subsystem2/1(Out1) -> Merge/3

== system CompleteEngineModel_turbo/Engine/Throttle  ==
  note: You are expected to implement your model here!
  p_im [Pa] : Inport
  pos [-] : Inport  Port=2
  p_bef,thr [Pa] : Inport  Port=3
  A_eff : Subsystem
  Divide : Product  Inputs=*/
  Divide1 : Product  Inputs=*/
  Product : Product  Inputs=3
  Product1 : Product
  Psi(PI) : Subsystem
  R : Constant  Value=R_air
  Sqrt : Sqrt  SaturateOnIntegerOverflow=on
  T_bef_thr : Constant  Value=mean(T_bef_thr)
  m_dot_at [kg/s]1 : Outport
  m_dot_at [kg/s] : Outport  Port=2
  wires:
  p_im [Pa]/1 -> Divide/1  "p_im"
  p_bef,thr [Pa]/1 -> Product/2, Divide/2  "p_bef_thr"
  pos [-]/1 -> A_eff/1(alpha)  "alpha"
  Divide/1 -> Psi(PI)/1(PI)
  A_eff/1(A_eff) -> Product/3
  Psi(PI)/1(Psi) -> Product/1  "Psi"
  Product/1 -> Divide1/1
  Divide1/1 -> m_dot_at [kg/s]1/1, m_dot_at [kg/s]/1
  R/1 -> Product1/1
  T_bef_thr/1 -> Product1/2
  Product1/1 -> Sqrt/1
  Sqrt/1 -> Divide1/2
